simulink model "DMC_Model"  (R2022b)
settings: Solver=FixedStepAuto  StartTime=0.0  StopTime=5.0  FixedStep=0.01  RelTol=1e-3
values from neighbouring files (symbols this model uses):
  Ks = 195    [Servo_calc_lq.m]    (also in Servo_calc_lq_d.m; servo_start.m)
  Ts = 0.86    [Servo_calc_lq.m]    (also in Servo_calc_lq_d.m; servo_start.m)
settings Model: Creator=artur  LastModifiedBy=artur

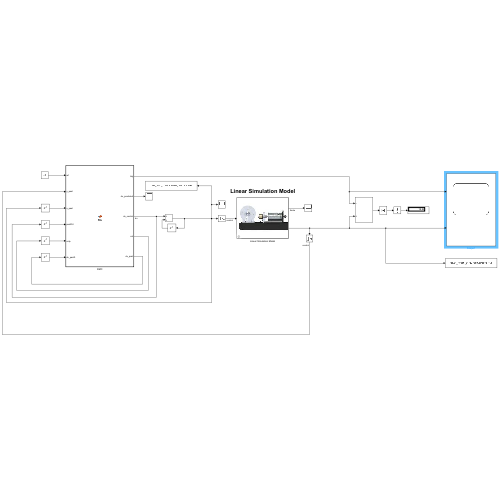
[thumbnail: Simulink's stored preview of the top-level diagram]
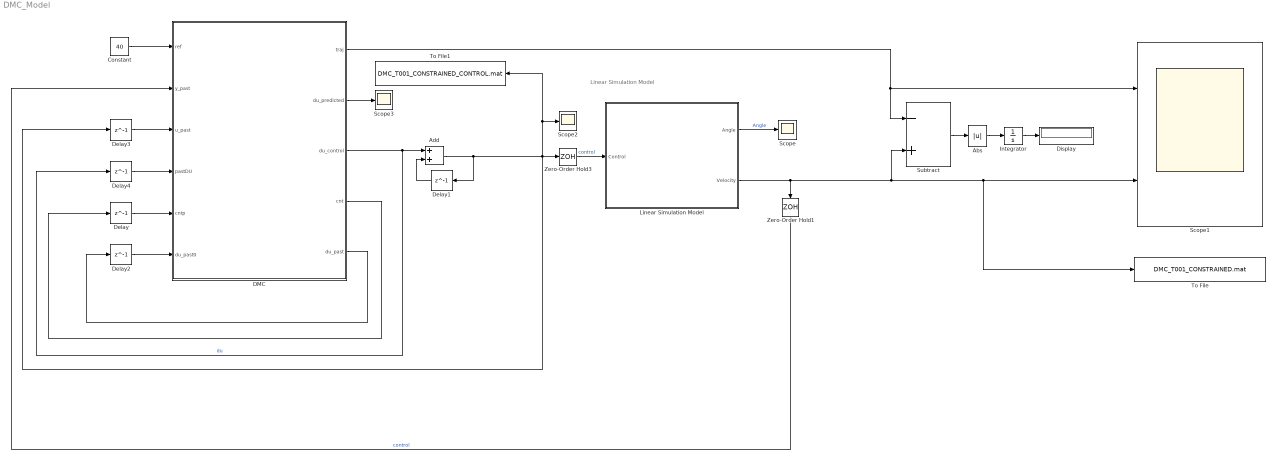
== system DMC_Model ==
  note: Linear Simulation Model
  Abs : Abs  SaturateOnIntegerOverflow=off
  Add : Sum
  Constant : Constant  Value=40
  DMC : MATLAB Function  TreatAsAtomicUnit=on
  Delay : Delay  DelayLength=1  InitialCondition=1
  Delay1 : Delay  DelayLength=1  InitialCondition=0
  Delay2 : Delay  DelayLength=1  InitialCondition=zeros(1,500-1)
  Delay3 : Delay  DelayLength=1  InitialCondition=0
  Delay4 : Delay  DelayLength=1  InitialCondition=0
  Display : Display
  Integrator : Integrator
  Linear Simulation Model : Subsystem  mask{x0=[0 0]}
      mask prompts: x0 "Initial conditions [angle vel]"
      mask Display: image(imread('Servo_m.JPG'))
  Scope : Scope
  Scope1 : Scope  NumInputPorts=2
  Scope2 : Scope
  Scope3 : Scope
  Subtract : Sum  Inputs=-+
  To File : ToFile  Filename=DMC_T001_CONSTRAINED.mat  SaveFormat=Timeseries
  To File1 : ToFile  Filename=DMC_T001_CONSTRAINED_CONTROL.mat  SaveFormat=Timeseries
  Zero-Order Hold1 : ZeroOrderHold  SampleTime=-1
  Zero-Order Hold3 : ZeroOrderHold  SampleTime=-1
  wires:
  Linear Simulation Model/1(Angle) -> Scope/1  "Angle"
  Add/1 -> Delay1/1, To File1/1, Scope2/1, Delay3/1, Zero-Order Hold3/1
  DMC/4(cnt) -> Delay/1
  Delay/1 -> DMC/5(cntp)
  Delay1/1 -> Add/2
  DMC/3(du_control) -> Add/1, Delay4/1  "du"
  DMC/2(du_predicted) -> Scope3/1
  Constant/1 -> DMC/1(ref)
  Delay3/1 -> DMC/3(u_past)
  Delay4/1 -> DMC/4(pastDU)
  DMC/1(traj) -> Scope1/1, Subtract/1
  Integrator/1 -> Display/1
  Abs/1 -> Integrator/1
  Subtract/1 -> Abs/1
  Linear Simulation Model/2(Velocity) -> Zero-Order Hold1/1, To File/1, Scope1/2, Subtract/2
  DMC/5(du_past) -> Delay2/1
  Delay2/1 -> DMC/6(du_past0)
  Zero-Order Hold3/1 -> Linear Simulation Model/1(Control)  "control"
  Zero-Order Hold1/1 -> DMC/2(y_past)  "control"

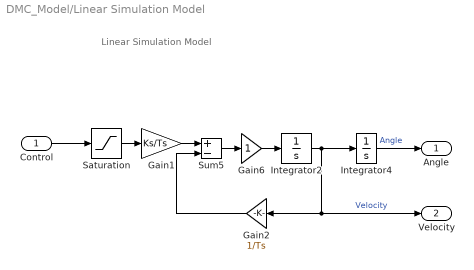
== system DMC_Model/Linear Simulation Model ==
  note: Linear Simulation Model
  Control : Inport
  Gain1 : Gain  Gain=Ks/Ts  SaturateOnIntegerOverflow=on  OutDataTypeStr=Inherit: Same as input  ParamDataTypeStr=Inherit: Same as input
  Gain2 : Gain  Gain=1/Ts  SaturateOnIntegerOverflow=on  OutDataTypeStr=Inherit: Same as input  ParamDataTypeStr=Inherit: Same as input
  Gain6 : Gain  SaturateOnIntegerOverflow=on  OutDataTypeStr=Inherit: Same as input  ParamDataTypeStr=Inherit: Same as input
  Integrator2 : Integrator  InitialCondition=x0(2)
  Integrator4 : Integrator  InitialCondition=x0(1)
  Saturation : Saturate  UpperLimit=1  LowerLimit=-1
  Sum5 : Sum  Inputs=+-  InputSameDT=on  SaturateOnIntegerOverflow=on  OutDataTypeStr=Inherit: Same as first input
  Angle : Outport  InitialOutput=0  VectorParamsAs1DForOutWhenUnconnected=off
  Velocity : Outport  Port=2  InitialOutput=0  VectorParamsAs1DForOutWhenUnconnected=off
  wires:
  Sum5/1 -> Gain6/1
  Gain2/1 -> Sum5/2
  Integrator2/1 -> Integrator4/1, Velocity/1, Gain2/1  "Velocity"
  Integrator4/1 -> Angle/1  "Angle"
  Gain6/1 -> Integrator2/1
  Control/1 -> Saturation/1
  Saturation/1 -> Gain1/1
  Gain1/1 -> Sum5/1

== matlab function DMC_Model/DMC ==
  data: traj output; du_predicted output; ref input; y_past input; u_past input; pastDU input; du_control output; cntp input; cnt output; du_past0 input; du_past output
function [traj,du_predicted, du_control,cnt,du_past] = fcn(ref,y_past,u_past,pastDU,cntp,du_past0)

cnt = cntp;
    
%Parametry
    ny = 500; %HORYZONT PREDYKCJI
    nu = 50; %HORYZONT STEROWANIA
    lambda = 1;
    D = 500;
    ograniczenie_wyjscia = false;
    
%Wektor przeszłych du
for i = 1:D-2
    du_past0(D-i) = du_past0(D-1-i);
end

du_past0(1) = pastDU;
du_past = du_past0;


% %Ustawienie ograniczeń dla optymalizatora 
    du_max = 0.1;
    du_min = -0.1;
    u_max = 0.6;
    u_min = -0.6;
    y_max = 42;
    y_min = -42;

%Trajektoria referencyjna, stała
Ts = 0.01; %PRÓBKOWANIE SYMULACJI
sim_time = 5; %CZAS SYMULACJI

traj_ub = ref*ones(1/Ts*sim_time/2,1);

traj_lb = -ref*ones(1/Ts*sim_time/2,1);

trajektoria = [traj_ub;traj_lb;-ref*ones(ny,1)];

ref = trajektoria(cnt:ny+cnt-1, 1);

cnt = cntp + 1;

traj = ref(1);

    
%Wyznaczenie macierzy predykcji
    
    [H,P] = dmc_predmat(ny,nu,D);
    Q = ones(ny,1);
    
%Prawo sterowania dla algorytmu z ograniczeniami
    S = H'*H + eye(nu)*lambda;
    S = (S + S')/2;
    f = H'*Q * y_past + H'*P * du_past - H' * ref;

%OGRANICZENIA
    if ograniczenie_wyjscia == true
        %OGRANICZENIA Z Y
        [C,dd,du,ddu,dy] = mpc_ograniczenia(du_max,du_min,u_max,u_min,y_max,y_min,nu,H,P,Q,D-1,1);
        dt = dd + du * u_past + ddu * du_past + dy*y_past;
    else
        %OGRANICZENIA BEZ Y
        [C, dd,du] = mpc_ograniczenia_bez_y(du_max,du_min,u_max,u_min,nu);
        dt = dd + du * u_past;
    end

    opts = optimoptions('quadprog','Algorithm','active-set');

    x0 = 1*eye(nu,1);

    du_predicted = quadprog(S,f,C,dt,[],[],[],[],x0,opts);

    du_control = du_predicted(1);

%Prawo sterowania dla algorytmu bez ograniczeń
% Pr = ( inv(H'*H+lambda*eye(nu)) ) * H';
% Nk = Pr*Q;
% Dk = Pr*P;
% 
% du_predicted = Pr * ref - Dk * du_past - Nk*y_past;
% du_control = du_predicted(1);

%Alternatywne prawo sterowania
% G = H;
% w = ref;
% f = Q *y_past + P * du_past;
% 
% du_predicted = inv(G' * G + lambda*eye(nu) ) * G' * (w - f);
% du_control = du_predicted(1);
